simulink model "DSSS_main"  (Simulink 9.3)
settings: Solver=ode45  StartTime=0.0  StopTime=inf  RelTol=1e-3  EnableMultiTasking=on
undefined symbols (not defined in the file or in its folder): doppler
libraries: dspindex x6, commchan3 x4, commfilt2 x3, commseqgen2 x2, commdigbbndam3 x2, dspbuff3 x2, commsink2 x1, commrandsrc2 x1, commutil2 x1
settings Model: Creator=Jinwoo Kim  LastModifiedBy=hwanju
settings DataIOCC: LimitDataPoints=on
settings OptimizationCC: ExpressionDepthLimit=2147483647  InitFltsAndDblsToZero=on
settings DebuggingCC: SaveWithParameterizedLinksMsg=none  SignalResolutionControl=TryResolveAllWithWarning  SolverPrmCheckMsg=warning  MultiTaskDSMMsg=warning  MultiTaskCondExecSysMsg=none  StateNameClashWarn=warning  SFExecutionAtInitializationDiag=warning
settings GRTTargetCC: TargetFcnLib=ansi_tfl_tmw.mat  GeneratePreprocessorConditionals=Disable all
settings CustomProperty: DataType=string  Value=0

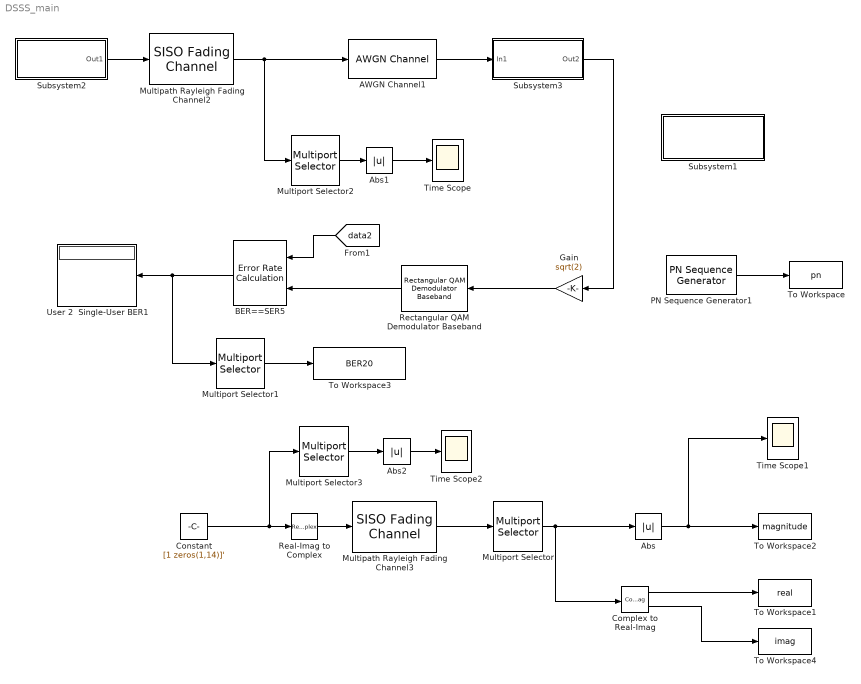
== system DSSS_main ==
  AWGN Channel1 : commchan3/AWGN Channel  InputProcessing=Columns as channels (frame based)  seed=67  noiseMode="Signal to noise ratio  (Eb/No)"  EbNodB=10  EsNodB=10  SNRdB=7  bitsPerSym=30  Ps=1  Tsym=1e-3  variance=1
      settings: SourceProductName=Communications Toolbox
  Abs : Abs
  Abs1 : Abs
  Abs2 : Abs
  BER==SER5 : commsink2/Error Rate Calculation  N=2  st_delay=0  cp_mode=Entire frame  subframe=[]  PMode=Port  WsName=ErrorVec  RsMode2=off  stop=off  numErr=100  maxBits=1e6
      settings: SourceProductName=Communications Toolbox
  Complex to Real-Imag : ComplexToRealImag
  Constant : Constant  Value=[1 zeros(1,14)]'  VectorParams1D=off  SampleTime=1  FramePeriod=1e-3
      settings: SamplingMode=Frame based
  Gain : Gain  Gain=sqrt(2)  SaturateOnIntegerOverflow=on
  Multipath Rayleigh Fading Channel2 : commchan3/SISO Fading Channel  InheritSampleRate=on  SampleRate=1  PathDelays="[0 1e-3/15  2e-3/15]"  AveragePathGains=[0 -3 -6]  NormalizePathGains=on  FadingDistribution=Rayleigh  KFactor=3  DirectPathDopplerShift=0  DirectPathInitialPhase=0  MaximumDopplerShift=10  DopplerSpectrum=doppler('Jakes')  ChannelInterpolationMethod=Polyphase  RandomStream=mt19937ar with seed  RandomNumGenerator=shr3cong  Seed=67  PathGainsOutputPort=off  ChannelFilterDelayOutputPort=off  SimulateUsing=Interpreted execution  Visualization=Off  PathsForDopplerDisplay=1  SamplesToDisplay=25%
      settings: SourceProductName=Communications Toolbox
  Multipath Rayleigh Fading Channel3 : commchan3/SISO Fading Channel  InheritSampleRate=on  SampleRate=1  PathDelays=[0]  AveragePathGains=[0]  NormalizePathGains=on  FadingDistribution=Rayleigh  KFactor=3  DirectPathDopplerShift=0  DirectPathInitialPhase=0  MaximumDopplerShift=10  DopplerSpectrum=doppler('Jakes')  ChannelInterpolationMethod=Polyphase  RandomStream=mt19937ar with seed  RandomNumGenerator=shr3cong  Seed=67  PathGainsOutputPort=off  ChannelFilterDelayOutputPort=off  SimulateUsing=Interpreted execution  Visualization=Off  PathsForDopplerDisplay=1  SamplesToDisplay=25%
      settings: SourceProductName=Communications Toolbox
  Multiport Selector{,1..3} (4 alike) : dspindex/Multiport Selector  rowsOrCols=Rows  idxCellArray={1}  idxErrMode=Clip Index
  PN Sequence Generator1 : commseqgen2/PN Sequence Generator  poly=[1 1 0 0 1]  ini_sta=[0 0 0 1]  outBitMaskSource=Dialog parameter  shift=3  outVarSiz=off  maxOutSizeMode=Dialog parameter  maxOutSize=[10 1]  Ts=1e-3  frameBased=off  sampPerFrame=1  reset=off  bitPackedOutputs=off  outDataType=double  numPackedBits=8  bitPackDataSigned=off  bitPackedOutDType=double
      settings: SourceProductName=Communications Toolbox  SourceProductBaseCode=CM
  Real-Imag to Complex : RealImagToComplex  Input=Real
  Rectangular QAM Demodulator Baseband : commdigbbndam3/Rectangular QAM Demodulator Baseband  M=4  OutType=Bit  DecType=Hard decision  VarSource=Dialog  Variance=1  Dec=Gray  Mapping=[0:15]  PowType=Min. distance between symbols  MinDist=2  AvgPow=1  PeakPow=1  Ph=0  outDtype1=double  outDtype2=double  derotateFactorWordLen=16  derotateFactorDataTypeStr=Inherit: Same word length as input  derotateFactorLastDataTypeStr=Inherit: Same word length as input  denormFactorWordLen=16  denormFactorDataTypeStr=Inherit: Same word length as input  denormFactorLastDataTypeStr=Inherit: Same word length as input  prodOutWordLen=32  prodOutOverflowMode=Wrap  prodOutRoundingMode=Floor  prodOutOvFlMode=off  prodOutOvFlModeLastStrValue=off  sumWordLen=32
      settings: SourceProductName=Communications Toolbox
  Subsystem1 : Subsystem
      mask Display: disp('Channel Estimation')
  Subsystem2 : Subsystem
      mask Display: disp('Tx')
  Subsystem3 : Subsystem
      mask Display: disp('Rx')
  Time Scope : Scope
  Time Scope1 : Scope
  Time Scope2 : Scope
  "To Workspace " : ToWorkspace  VariableName=pn  SampleTime=-1
      settings: MaxDataPoints=30  Save2DSignal=2-D array (concatenate along first dimension)
  To Workspace1 : ToWorkspace  VariableName=real  SampleTime=-1
      settings: Save2DSignal=2-D array (concatenate along first dimension)
  "To Workspace2 " : ToWorkspace  VariableName=magnitude  SampleTime=-1
      settings: Save2DSignal=2-D array (concatenate along first dimension)
  To Workspace3 : ToWorkspace  VariableName=BER20  SampleTime=-1
      settings: MaxDataPoints=1
  "To Workspace4 " : ToWorkspace  VariableName=imag  SampleTime=-1
      settings: Save2DSignal=2-D array (concatenate along first dimension)
  User 2  Single-User BER1 : Display
  wires:
  AWGN Channel1/1 -> Subsystem3/1(In1)
  Subsystem2/1(Out1) -> Multipath Rayleigh Fading Channel2/1
  Gain/1 -> Rectangular QAM Demodulator Baseband/1
  [data2] -> BER==SER5/1
  Rectangular QAM Demodulator Baseband/1 -> BER==SER5/2
  BER==SER5/1 -> User 2  Single-User BER1/1, Multiport Selector1/1
  Subsystem3/1(Out2) -> Gain/1
  Constant/1 -> Real-Imag to Complex/1, Multiport Selector3/1
  Real-Imag to Complex/1 -> Multipath Rayleigh Fading Channel3/1
  Multipath Rayleigh Fading Channel3/1 -> Multiport Selector/1
  Multiport Selector/1 -> Abs/1, Complex to Real-Imag/1
  Multiport Selector1/1 -> To Workspace3/1
  PN Sequence Generator1/1 -> "To Workspace "/1
  Abs/1 -> "To Workspace2 "/1, Time Scope1/1
  Complex to Real-Imag/1 -> To Workspace1/1
  Complex to Real-Imag/2 -> "To Workspace4 "/1
  Multipath Rayleigh Fading Channel2/1 -> AWGN Channel1/1, Multiport Selector2/1
  Multiport Selector2/1 -> Abs1/1
  Abs1/1 -> Time Scope/1
  Multiport Selector3/1 -> Abs2/1
  Abs2/1 -> Time Scope2/1

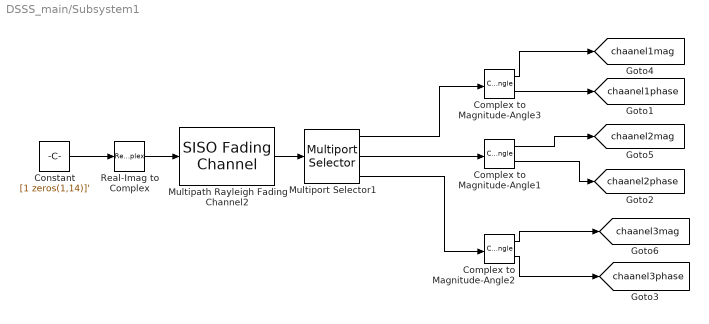
== system DSSS_main/Subsystem1 ==
  Complex to Magnitude-Angle1 : ComplexToMagnitudeAngle
  Complex to Magnitude-Angle2 : ComplexToMagnitudeAngle
  Complex to Magnitude-Angle3 : ComplexToMagnitudeAngle
  Constant : Constant  Value=[1 zeros(1,14)]'  VectorParams1D=off  SampleTime=1  FramePeriod=1e-3
      settings: SamplingMode=Frame based
  Multipath Rayleigh Fading Channel2 : commchan3/SISO Fading Channel  InheritSampleRate=on  SampleRate=1  PathDelays="[0 1e-3/15  2e-3/15]"  AveragePathGains=[0 -3 -6]  NormalizePathGains=on  FadingDistribution=Rayleigh  KFactor=3  DirectPathDopplerShift=0  DirectPathInitialPhase=0  MaximumDopplerShift=10  DopplerSpectrum=doppler('Jakes')  ChannelInterpolationMethod=Polyphase  RandomStream=mt19937ar with seed  RandomNumGenerator=shr3cong  Seed=67  PathGainsOutputPort=off  ChannelFilterDelayOutputPort=off  SimulateUsing=Interpreted execution  Visualization=Off  PathsForDopplerDisplay=1  SamplesToDisplay=25%
      settings: SourceProductName=Communications Toolbox
  Multiport Selector1 : dspindex/Multiport Selector  rowsOrCols=Rows  idxCellArray={1,2,3}  idxErrMode=Clip Index
  Real-Imag to Complex : RealImagToComplex  Input=Real
  tag scope: chaanel1mag=global, chaanel1phase=global, chaanel2mag=global, chaanel2phase=global, chaanel3mag=global, chaanel3phase=global
  wires:
  Constant/1 -> Real-Imag to Complex/1
  Real-Imag to Complex/1 -> Multipath Rayleigh Fading Channel2/1
  Multipath Rayleigh Fading Channel2/1 -> Multiport Selector1/1
  Multiport Selector1/1 -> Complex to Magnitude-Angle3/1
  Multiport Selector1/2 -> Complex to Magnitude-Angle1/1
  Multiport Selector1/3 -> Complex to Magnitude-Angle2/1
  Complex to Magnitude-Angle3/2 -> [chaanel1phase]
  Complex to Magnitude-Angle1/2 -> [chaanel2phase]
  Complex to Magnitude-Angle2/2 -> [chaanel3phase]
  Complex to Magnitude-Angle3/1 -> [chaanel1mag]
  Complex to Magnitude-Angle2/1 -> [chaanel3mag]
  Complex to Magnitude-Angle1/1 -> [chaanel2mag]

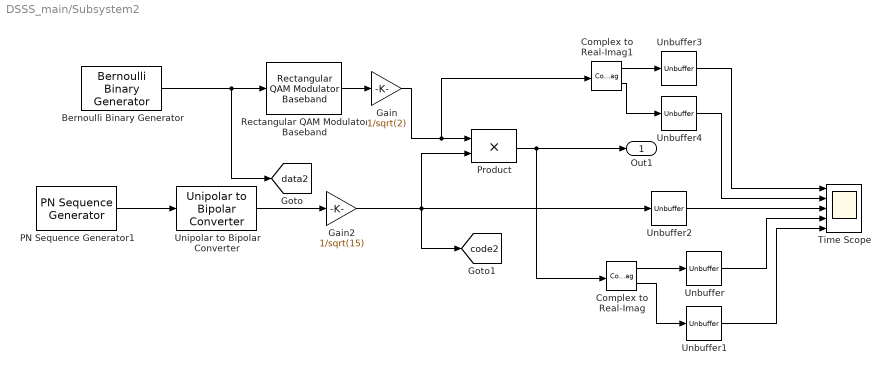
== system DSSS_main/Subsystem2 ==
  Bernoulli Binary Generator : commrandsrc2/Bernoulli Binary Generator  P=0.5  seed=61  Ts=1e-3/2  frameBased=on  sampPerFrame=2  orient=off  outDataType=double
      settings: SourceProductName=Communications Toolbox  SourceProductBaseCode=CM
  Complex to Real-Imag : ComplexToRealImag
  Complex to Real-Imag1 : ComplexToRealImag
  Gain : Gain  Gain=1/sqrt(2)  SaturateOnIntegerOverflow=on  OutDataTypeStr=Inherit: Same as input  ParamDataTypeStr=Inherit: Same as input
  Gain2 : Gain  Gain=1/sqrt(15)  SaturateOnIntegerOverflow=on  OutDataTypeStr=Inherit: Same as input  ParamDataTypeStr=Inherit: Same as input
  PN Sequence Generator1 : commseqgen2/PN Sequence Generator  poly=[1 1 0 0 1]  ini_sta=[0 0 0 1]  outBitMaskSource=Dialog parameter  shift=0  outVarSiz=off  maxOutSizeMode=Dialog parameter  maxOutSize=[10 1]  Ts=1e-3/15  frameBased=on  sampPerFrame=15  reset=off  bitPackedOutputs=off  outDataType=double  numPackedBits=8  bitPackDataSigned=off  bitPackedOutDType=double
      settings: SourceProductName=Communications Toolbox  SourceProductBaseCode=CM
  Product : Product  SaturateOnIntegerOverflow=on  InputSameDT=on  OutDataTypeStr=Inherit: Same as first input
  Rectangular QAM Modulator Baseband : commdigbbndam3/Rectangular QAM Modulator Baseband  M=4  InType=Bit  Enc=Gray  Mapping=[0:15]  PowType=Min. distance between symbols  MinDist=2  AvgPow=1  PeakPow=1  Ph=0  outDtype=double  outWordLen=16  outUDDataType=sfix(16)  outFracLenMode=Best precision  outFracLen=15  outDataTypeStr=double  outLastDataTypeStr=double
      settings: SourceProductName=Communications Toolbox
  Time Scope : Scope  NumInputPorts=5
  Unbuffer{,1..4} (5 alike) : Unbuffer
  Unipolar to Bipolar Converter : commutil2/Unipolar to Bipolar Converter  M=2  polarity=Positive  dataType=Same as input
      settings: SourceProductName=Communications Toolbox
  Out1 : Outport
  tag scope: code2=global, data2=global
  wires:
  Gain/1 -> Product/1, Complex to Real-Imag1/1
  Gain2/1 -> Product/2, Unbuffer2/1, [code2]
  Product/1 -> Out1/1, Complex to Real-Imag/1
  Unipolar to Bipolar Converter/1 -> Gain2/1
  Rectangular QAM Modulator Baseband/1 -> Gain/1
  Bernoulli Binary Generator/1 -> Rectangular QAM Modulator Baseband/1, [data2]
  PN Sequence Generator1/1 -> Unipolar to Bipolar Converter/1
  Complex to Real-Imag/1 -> Unbuffer/1
  Complex to Real-Imag/2 -> Unbuffer1/1
  Unbuffer2/1 -> Time Scope/3
  Complex to Real-Imag1/1 -> Unbuffer3/1
  Complex to Real-Imag1/2 -> Unbuffer4/1
  Unbuffer3/1 -> Time Scope/1
  Unbuffer4/1 -> Time Scope/2
  Unbuffer/1 -> Time Scope/4
  Unbuffer1/1 -> Time Scope/5

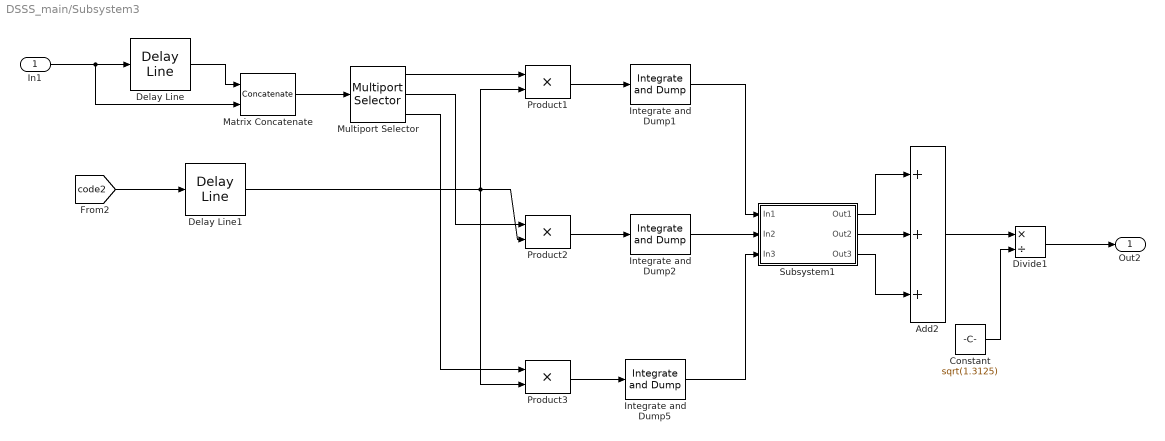
== system DSSS_main/Subsystem3 ==
  In1 : Inport
  Add2 : Sum  Inputs=+++
  Constant : Constant  Value=sqrt(1.3125)
  Delay Line : dspbuff3/Delay Line  siz=15  ic=0  directfeed=off  enable_output=off  hold_output=off  OutputFrames=on
      settings: SourceProductName=DSP System Toolbox  SourceProductBaseCode=DS
  Delay Line1 : dspbuff3/Delay Line  siz=15  ic=0  directfeed=off  enable_output=off  hold_output=off  OutputFrames=on
      settings: SourceProductName=DSP System Toolbox  SourceProductBaseCode=DS
  Divide1 : Product  Inputs=*/
  Integrate and Dump1 : commfilt2/Integrate and Dump  obssamples=15  offsetsamples=0  nodump=off  roundingMode=Floor  overflowMode=off  outputDataTypeStr=Inherit: Same as accumulator  outputLastDataTypeStr=Inherit: Same as accumulator
      settings: SourceProductName=Communications Toolbox
  Integrate and Dump2 : commfilt2/Integrate and Dump  obssamples=15  offsetsamples=0  nodump=off  roundingMode=Floor  overflowMode=off  outputDataTypeStr=Inherit: Same as accumulator  outputLastDataTypeStr=Inherit: Same as accumulator
      settings: SourceProductName=Communications Toolbox
  Integrate and Dump5 : commfilt2/Integrate and Dump  obssamples=15  offsetsamples=0  nodump=off  roundingMode=Floor  overflowMode=off  outputDataTypeStr=Inherit: Same as accumulator  outputLastDataTypeStr=Inherit: Same as accumulator
      settings: SourceProductName=Communications Toolbox
  Matrix Concatenate : Concatenate  Mode=Multidimensional array
  Multiport Selector : dspindex/Multiport Selector  rowsOrCols=Rows  idxCellArray={1:15, 2:16, 3:17}  idxErrMode=Clip Index
  Product1 : Product  SaturateOnIntegerOverflow=on  InputSameDT=on  OutDataTypeStr=Inherit: Same as first input
  Product2 : Product  SaturateOnIntegerOverflow=on  InputSameDT=on  OutDataTypeStr=Inherit: Same as first input
  Product3 : Product  SaturateOnIntegerOverflow=on  InputSameDT=on  OutDataTypeStr=Inherit: Same as first input
  Subsystem1 : Subsystem
      mask Display: disp('MRC Combining')
  Out2 : Outport
  wires:
  Product1/1 -> Integrate and Dump1/1
  Product2/1 -> Integrate and Dump2/1
  [code2] -> Delay Line1/1
  Delay Line/1 -> Matrix Concatenate/1
  Matrix Concatenate/1 -> Multiport Selector/1
  Multiport Selector/1 -> Product1/1
  Multiport Selector/2 -> Product2/1
  Delay Line1/1 -> Product2/2, Product1/2, Product3/2
  In1/1 -> Delay Line/1, Matrix Concatenate/2
  Multiport Selector/3 -> Product3/1
  Product3/1 -> Integrate and Dump5/1
  Integrate and Dump1/1 -> Subsystem1/1(In1)
  Integrate and Dump2/1 -> Subsystem1/2(In2)
  Integrate and Dump5/1 -> Subsystem1/3(In3)
  Subsystem1/1(Out1) -> Add2/1
  Add2/1 -> Divide1/1
  Divide1/1 -> Out2/1
  Constant/1 -> Divide1/2
  Subsystem1/2(Out2) -> Add2/2
  Subsystem1/3(Out3) -> Add2/3

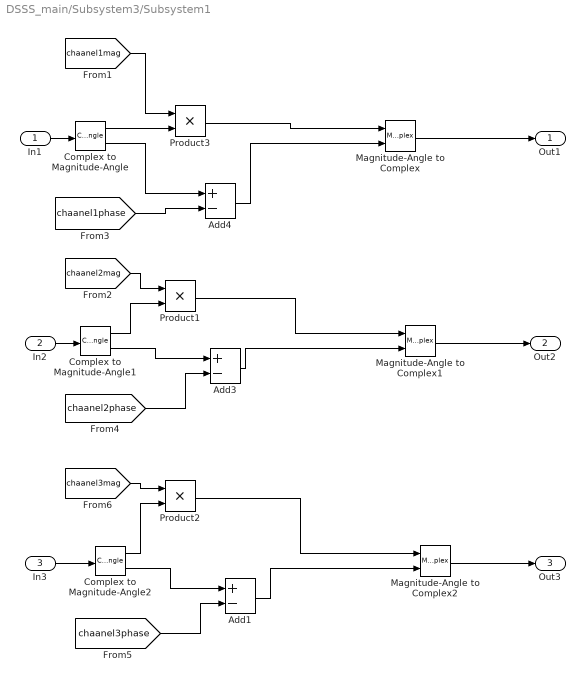
== system DSSS_main/Subsystem3/Subsystem1 ==
  In1 : Inport
  In2 : Inport  Port=2
  In3 : Inport  Port=3
  Add1 : Sum  Inputs=+-
  Add3 : Sum  Inputs=+-
  Add4 : Sum  Inputs=+-
  Complex to Magnitude-Angle : ComplexToMagnitudeAngle
  Complex to Magnitude-Angle1 : ComplexToMagnitudeAngle
  Complex to Magnitude-Angle2 : ComplexToMagnitudeAngle
  Magnitude-Angle to Complex : MagnitudeAngleToComplex
  Magnitude-Angle to Complex1 : MagnitudeAngleToComplex
  Magnitude-Angle to Complex2 : MagnitudeAngleToComplex
  Product1 : Product  RndMeth=Zero
  Product2 : Product  RndMeth=Zero
  Product3 : Product  RndMeth=Zero
  Out1 : Outport
  Out2 : Outport  Port=2
  Out3 : Outport  Port=3
  wires:
  [chaanel2phase] -> Add3/2
  [chaanel3phase] -> Add1/2
  Complex to Magnitude-Angle/2 -> Add4/1
  Complex to Magnitude-Angle2/2 -> Add1/1
  Add4/1 -> Magnitude-Angle to Complex/2
  Add3/1 -> Magnitude-Angle to Complex1/2
  Add1/1 -> Magnitude-Angle to Complex2/2
  Complex to Magnitude-Angle1/2 -> Add3/1
  In1/1 -> Complex to Magnitude-Angle/1
  In2/1 -> Complex to Magnitude-Angle1/1
  In3/1 -> Complex to Magnitude-Angle2/1
  Magnitude-Angle to Complex/1 -> Out1/1
  Magnitude-Angle to Complex1/1 -> Out2/1
  Magnitude-Angle to Complex2/1 -> Out3/1
  [chaanel1phase] -> Add4/2
  [chaanel2mag] -> Product1/1
  Complex to Magnitude-Angle1/1 -> Product1/2
  [chaanel3mag] -> Product2/1
  Complex to Magnitude-Angle2/1 -> Product2/2
  Product2/1 -> Magnitude-Angle to Complex2/1
  Product1/1 -> Magnitude-Angle to Complex1/1
  [chaanel1mag] -> Product3/1
  Complex to Magnitude-Angle/1 -> Product3/2
  Product3/1 -> Magnitude-Angle to Complex/1
